simulink model "HITL"  (R2017b)
settings: Solver=FixedStepDiscrete  StartTime=0.0  StopTime=inf  FixedStep=0.1  RelTol=1e-3
InitFcn:
  | initHITL
libraries: etargetslib x1, dspnetwork x1
settings Model: Creator=b6034940  LastModifiedBy=fahim
settings CodeAppCC: StateflowObjectComments=on

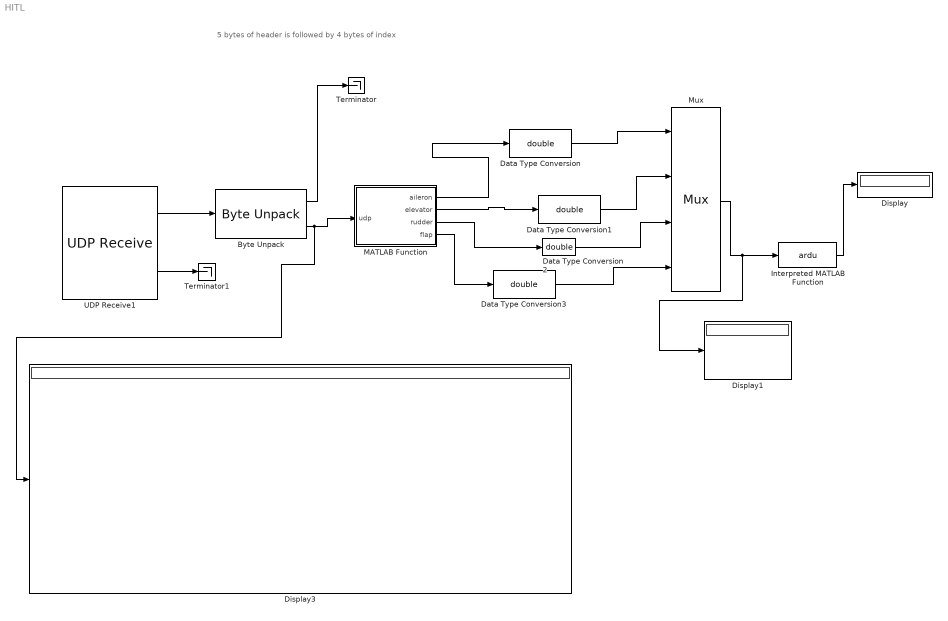
== system HITL ==
  note: 5 bytes of header is followed by 4 bytes of index
  Byte Unpack : etargetslib/Byte Unpack  dimensions={5,[9,8]}  datatypes={'uint8','single'}  byteAlign=1
  Data Type Conversion{,1..3} (4 alike) : DataTypeConversion  OutDataTypeStr=double
  Display : Display
  Display1 : Display
  Display3 : Display
  Interpreted MATLAB Function : MATLABFcn  MATLABFcn=ardu
  MATLAB Function : MATLAB Function  TreatAsAtomicUnit=on
  Mux : Mux
  Terminator : Terminator
  Terminator1 : Terminator
  UDP Receive1 : dspnetwork/UDP Receive  localURL='0.0.0.0'  localPort=49001  remoteURL='127.0.0.1'  remotePort=-1  recvBufferSize=8192  dims=293  signalDatatype=uint8  isVarSize=off  showBlockingTime=off  blockingTime=0  sampletime=inf  blockPlatform=[]
      settings: SourceProductName=DSP System Toolbox  SourceProductBaseCode=DS
  wires:
  Byte Unpack/2 -> Display3/1, MATLAB Function/1(udp)
  MATLAB Function/1(aileron) -> Data Type Conversion/1
  MATLAB Function/2(elevator) -> Data Type Conversion1/1
  UDP Receive1/2 -> Terminator1/1
  UDP Receive1/1 -> Byte Unpack/1
  Byte Unpack/1 -> Terminator/1
  MATLAB Function/3(rudder) -> Data Type Conversion2/1
  Interpreted MATLAB Function/1 -> Display/1
  Data Type Conversion/1 -> Mux/1
  Data Type Conversion1/1 -> Mux/2
  Data Type Conversion2/1 -> Mux/3
  Mux/1 -> Display1/1, Interpreted MATLAB Function/1
  MATLAB Function/4(flap) -> Data Type Conversion3/1
  Data Type Conversion3/1 -> Mux/4

== matlab function HITL/MATLAB Function ==
  data: udp input; aileron output; elevator output; rudder output; flap output
function [aileron, elevator, rudder, flap] = extract(udp)
% global a
% global s
% a = arduino
% s = servo(a,'D6')

coder.extrinsic('round');

elevator = udp(2,1); % first packet 2nd value
elevator = round(elevator,1);

aileron = udp (3,1);
aileron = round(aileron,1);

rudder = udp (4,1);
rudder = round(rudder,1);
rudder = -1*rudder;

flap = udp(6,2);
flap = round(flap,1);

uu = [elevator, aileron, rudder, flap];

end
